simulink model "QuarterCar_2DoF_Model_v2"  (R2020b)
settings: Solver=VariableStepAuto  StartTime=0.0  StopTime=200  RelTol=1e-3
libraries: simulink x1
settings Model: Creator=ocwar  LastModifiedBy=ocwar

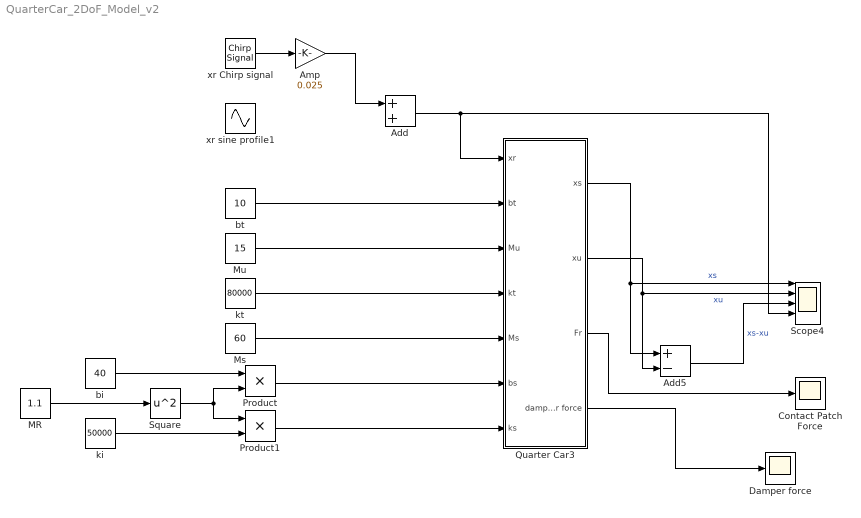
== system QuarterCar_2DoF_Model_v2 ==
  Add : Sum
  Add5 : Sum  Inputs=+-
  Amp : Gain  Gain=0.025
  Contact Patch Force : Scope
  Damper force : Scope
  MR : Constant  Value=1.1
  Ms : Constant  Value=60
  Mu : Constant  Value=15
  Product : Product
  Product1 : Product
  Quarter Car3 : Subsystem
  Scope4 : Scope  NumInputPorts=5
  Square : Math  Operator=square  SaturateOnIntegerOverflow=on
  bi : Constant  Value=40
  bt : Constant  Value=10
  ki : Constant  Value=50000
  kt : Constant  Value=80000
  xr Chirp signal : simulink/Sources/Chirp Signal  f1=0  T=200  f2=20
  xr sine profile1 : Sin  Amplitude=0.025  Frequency=5*2*pi  SampleTime=0
  wires:
  Quarter Car3/2(xu) -> Add5/2, Scope4/2  "xu"
  Quarter Car3/1(xs) -> Add5/1, Scope4/1  "xs"
  Add5/1 -> Scope4/3  "xs-xu"
  Quarter Car3/3(Fr) -> Contact Patch Force/1
  Mu/1 -> Quarter Car3/3(Mu)
  bt/1 -> Quarter Car3/2(bt)
  kt/1 -> Quarter Car3/4(kt)
  Ms/1 -> Quarter Car3/5(Ms)
  MR/1 -> Square/1
  Square/1 -> Product1/1, Product/2
  bi/1 -> Product/1
  Product1/1 -> Quarter Car3/7(ks)
  ki/1 -> Product1/2
  Add/1 -> Quarter Car3/1(xr), Scope4/4
  xr Chirp signal/1 -> Amp/1
  Quarter Car3/4(damper force) -> Damper force/1
  Product/1 -> Quarter Car3/6(bs)
  Amp/1 -> Add/1

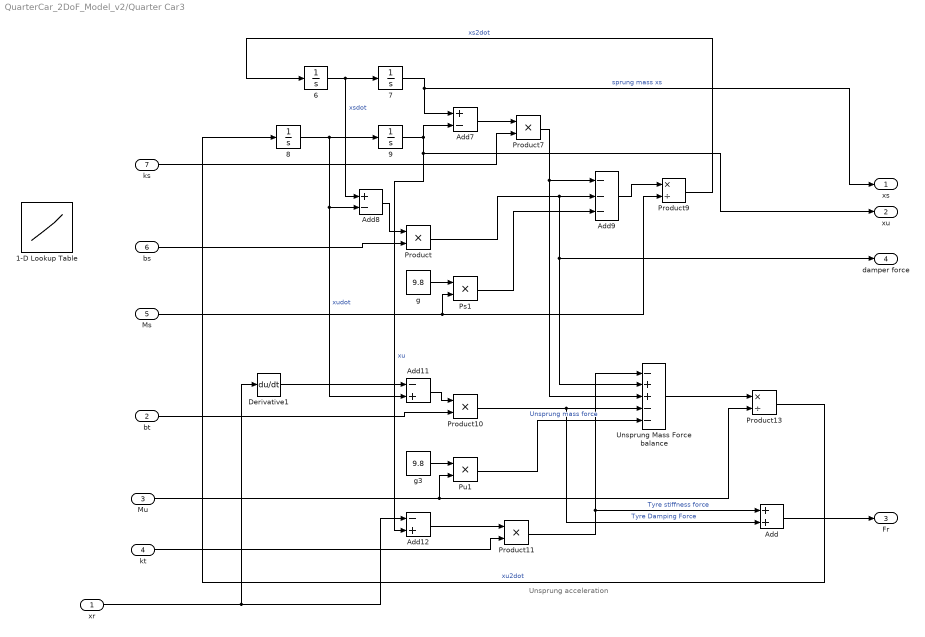
== system QuarterCar_2DoF_Model_v2/Quarter Car3 ==
  note: Unsprung acceleration
  xr : Inport
  bt : Inport  Port=2
  Mu : Inport  Port=3
  kt : Inport  Port=4
  Ms : Inport  Port=5
  bs : Inport  Port=6
  ks : Inport  Port=7
  1-D Lookup Table : Lookup_n-D  NumberOfTableDimensions=1  BreakpointsForDimension1=|  Table=|  InternalRulePriority=Speed  RndMeth=Simplest  InputSameDT=on
      BreakpointsForDimension1=|
      | [-0.225644916540091,
      | 26.0597193850446,
      | 89.0074586700638,
      | 270.404726303712
      | ,346.915511426249
      | ,449.375140194057]
      Table=|
      | [0.000200495672698680,
      | 0.00100247836349333,
      | 0.0164406451612903,
      | 0.0499234225019670,
      | 0.102453288749017,
      | 0.253827521636507]
  {6..9} (4 alike) : Integrator
  Add : Sum
  Add11 : Sum  Inputs=-+
  Add12 : Sum  Inputs=-+
  Add7 : Sum  Inputs=+-
  Add8 : Sum  Inputs=+-
  Add9 : Sum  Inputs=---
  Derivative1 : Derivative
  Product{,7,10..11} (4 alike) : Product
  Product13 : Product  Inputs=*/
  Product9 : Product  Inputs=*/
  Ps1 : Product
  Pu1 : Product
  Unsprung Mass Force balance : Sum  Inputs=-++--
  g : Constant  Value=9.8
  g3 : Constant  Value=9.8
  xs : Outport
  xu : Outport  Port=2
  Fr : Outport  Port=3
  damper force : Outport  Port=4
  wires:
  g/1 -> Ps1/1
  g3/1 -> Pu1/1
  Ps1/1 -> Add9/3
  Unsprung Mass Force balance/1 -> Product13/1
  Mu/1 -> Product13/2, Pu1/2
  Product11/1 -> Unsprung Mass Force balance/1, Add/1  "Tyre stiffness force"
  Add12/1 -> Product11/1
  kt/1 -> Product11/2
  xr/1 -> Add12/1, Derivative1/1
  Pu1/1 -> Unsprung Mass Force balance/5  "Unsprung mass force"
  Add11/1 -> Product10/1
  bt/1 -> Product10/2
  Derivative1/1 -> Add11/1
  Ms/1 -> Product9/2, Ps1/2
  Add9/1 -> Product9/1
  Product7/1 -> Unsprung Mass Force balance/3, Add9/1
  ks/1 -> Product7/2
  Add7/1 -> Product7/1
  9/1 -> Add12/2, xu/1, Add7/2  "xu"
  Product13/1 -> 8/1  "xu2dot"
  8/1 -> 9/1, Add11/2, Add8/2  "xudot"
  7/1 -> Add7/1, xs/1  "sprung mass xs"
  Product9/1 -> 6/1  "xs2dot"
  6/1 -> 7/1, Add8/1  "xsdot"
  Add/1 -> Fr/1
  Product10/1 -> Add/2, Unsprung Mass Force balance/4  "Tyre Damping Force"
  Add8/1 -> Product/1
  bs/1 -> Product/2
  Product/1 -> damper force/1, Unsprung Mass Force balance/2, Add9/2
